simulink model "MinSegShield_Demo_M2V3"  (R2015a)
settings: Solver=FixedStepDiscrete  SolverMode=SingleTasking  StartTime=0.0  StopTime=inf  FixedStep=.03  RelTol=1e-3
libraries: MinSegLibrary_M2V3 x11, arduinolib x5, RASPlib x1
settings Model: SimulationMode=external  ExtModeTrigDuration=2  Creator=Alec  LastModifiedBy=hurstj
settings OptimizationCC: ExpressionDepthLimit=2147483647  OptimizeModelRefInitCode=on  LifeSpan=1
settings DebuggingCC: UnderspecifiedInitializationDetection=Classic  MergeDetectMultiDrivingBlocksExec=none  StateNameClashWarn=warning
settings HardwareCC: ProdBitPerInt=16  ProdBitPerPointer=8  ProdIntDivRoundTo=Zero  ProdEndianess=LittleEndian  ProdWordSize=8  ProdHWDeviceType=Atmel->AVR
settings RTWCC: SystemTargetFile=realtime.tlc  GenerateMakefile=off  TemplateMakefile=realtime.tmf  Description=Real-Time Toolbox  RTWVerbose=off
settings CodeAppCC: MangleLength=10  CustomSymbolStrType=$N$R$M  InternalIdentifier=Classic
settings ERTTargetCC: CombineOutputUpdateFcns=off  ExtMode=on  ExtModeTransport=3  ExtModeMexArgs=0 82 115200  ERTSrcFileBannerTemplate=realtime_code_template.cgt  ERTHdrFileBannerTemplate=realtime_code_template.cgt  ERTDataSrcFileTemplate=realtime_code_template.cgt  ERTDataHdrFileTemplate=realtime_code_template.cgt  ERTCustomFileTemplate=realtime_file_process.tlc

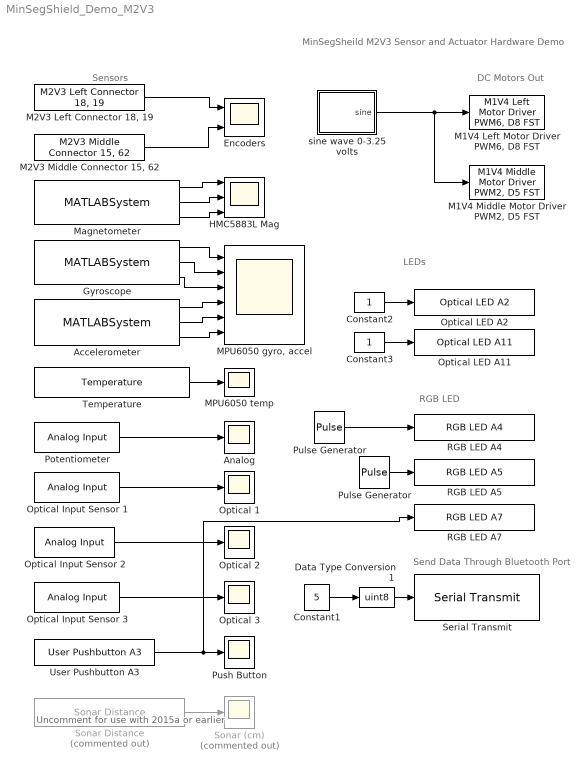
== system MinSegShield_Demo_M2V3 ==
  note: Send Data Through Bluetooth Port
  note: DC Motors Out
  note: Sensors
  note: MinSegSheild M2V3 Sensor and Actuator
      | Hardware Demo
  note: LEDs
  note: RGB LED
  note: Uncomment for use with 2015a or earlier
  Accelerometer : MATLABSystem  System=soMPU6050Accel  SimulateUsing=Code generation
      mask Type: soMPU6050Accel
      mask Display:
      | disp('soMPU6050Accel');
      | port_label('output',1,'xaccel');
      | port_label('output',2,'yaccel');
      | port_label('output',3,'zaccel');
  Analog : Scope
      settings: TimeRange=30  YMin=0  YMax=1000  SaveName=ScopeData6
  Constant1 : Constant  Value=5  SampleTime=-1
  Constant2 : Constant  SampleTime=-1
  Constant3 : Constant  SampleTime=-1
  Data Type Conversion1 : DataTypeConversion  OutDataTypeStr=uint8
  Encoders : Scope  NumInputPorts=2
      settings: TimeRange=20  YMin=-200~-25  YMax=700~250
  Gyroscope : MATLABSystem  System=soMPU6050Gyro  DLPFmode=0
      mask Type: soMPU6050Gyro
      mask Display:
      | disp('soMPU6050Gyro');
      | port_label('output',1,'xvel');
      | port_label('output',2,'yvel');
      | port_label('output',3,'zvel');
  HMC5883L Mag : Scope  NumInputPorts=3
      settings: TimeRange=10  YMin=100~-90~25  YMax=175~30~200  SaveName=ScopeData7
  "M1V4 Left Motor Driver PWM6, D8 FST" : MinSegLibrary_M2V3/M1V4 Left Motor Driver PWM6, D8 FST  Vsupply=3.25
  "M1V4 Middle Motor Driver PWM2, D5 FST" : MinSegLibrary_M2V3/M1V4 Middle Motor Driver PWM2, D5 FST  Vsupply=3.25
  "M2V3 Left Connector 18, 19" : MinSegLibrary_M2V3/M2V3 Left Connector 18, 19  Encoder=1  PinA=19  PinB=18  PWMFSelect=1  PWMTimer=3
  "M2V3 Middle Connector 15, 62" : MinSegLibrary_M2V3/M2V3 Middle Connector 15, 62  Encoder=3  PinA=15  PinB=62  PWMFSelect=1  PWMTimer=3
  "MPU6050 gyro, accel" : Scope  NumInputPorts=6
      settings: TimeRange=10  YMin=-650~-300~-275~100~-400~6000  YMax=-475~-75~-125~800~200~8000
  MPU6050 temp : Scope
      settings: TimeRange=30  YMin=-3750  YMax=-1750  SaveName=ScopeData9
  Magnetometer : MATLABSystem  System=soHMC5883L  SimulateUsing=Code generation
      mask Type: soHMC5883L
      mask Display:
      | disp('soHMC5883L');
      | port_label('output',1,'xmag');
      | port_label('output',2,'ymag');
      | port_label('output',3,'zmag');
  Optical 1 : Scope
      settings: TimeRange=30  YMin=0  YMax=1000  SaveName=ScopeData4
  Optical 2 : Scope
      settings: TimeRange=30  YMin=0  YMax=1000  SaveName=ScopeData3
  Optical 3 : Scope
      settings: TimeRange=30  YMin=0  YMax=1000  SaveName=ScopeData5
  Optical Input Sensor 1 : arduinolib/Analog Input  pinNumber=10  sampleTime=-1  blockPlatform=arduino
  Optical Input Sensor 2 : arduinolib/Analog Input  pinNumber=1  sampleTime=-1  blockPlatform=arduino
  Optical Input Sensor 3 : arduinolib/Analog Input  pinNumber=9  sampleTime=-1  blockPlatform=arduino
  Optical LED A11 : MinSegLibrary_M2V3/Optical LED A11  Pin=11
  Optical LED A2 : MinSegLibrary_M2V3/Optical LED A2  Pin=2
  Potentiometer : arduinolib/Analog Input  pinNumber=0  sampleTime=-1  blockPlatform=arduino
  Pulse Generator : DiscretePulseGenerator  PulseType=Time based  Period=9  PulseWidth=50
  "Pulse Generator " : DiscretePulseGenerator  PulseType=Time based  Period=6  PulseWidth=50
  Push Button : Scope
      settings: TimeRange=30  YMin=0.95  YMax=1.05  SaveName=ScopeData8
  RGB LED A4 : MinSegLibrary_M2V3/RGB LED A4  Pin=4
  RGB LED A5 : MinSegLibrary_M2V3/RGB LED A5  Pin=5
  "RGB LED A7 " : MinSegLibrary_M2V3/RGB LED A7   Pin=7
  Serial Transmit : arduinolib/Serial Transmit  portNumber=2  blockPlatform=arduino
  Sonar (cm) : Scope  Commented=on
      settings: TimeRange=10  YMin=0  YMax=175  SaveName=ScopeData2
  Sonar Distance : MinSegLibrary_M2V3/Sonar Distance  Commented=on  TrigPin=12  EchoPin=11
  Temperature : RASPlib/Temperature  SimulateUsing=Code generation
  User Pushbutton A3 : MinSegLibrary_M2V3/User Pushbutton A3  Pin=3
  sine wave 0-3.25 volts : Subsystem
  wires:
  "M2V3 Left Connector 18, 19"/1 -> Encoders/1
  "M2V3 Middle Connector 15, 62"/1 -> Encoders/2
  Sonar Distance/1 -> Sonar (cm)/1
  Optical Input Sensor 1/1 -> Optical 1/1
  Constant1/1 -> Data Type Conversion1/1
  Data Type Conversion1/1 -> Serial Transmit/1
  Optical Input Sensor 2/1 -> Optical 2/1
  Optical Input Sensor 3/1 -> Optical 3/1
  Potentiometer/1 -> Analog/1
  Magnetometer/2 -> HMC5883L Mag/2
  Magnetometer/3 -> HMC5883L Mag/3
  Gyroscope/1 -> "MPU6050 gyro, accel"/1
  Gyroscope/2 -> "MPU6050 gyro, accel"/2
  Gyroscope/3 -> "MPU6050 gyro, accel"/3
  Accelerometer/3 -> "MPU6050 gyro, accel"/6
  Magnetometer/1 -> HMC5883L Mag/1
  sine wave 0-3.25 volts/1(sine) -> "M1V4 Middle Motor Driver PWM2, D5 FST"/1, "M1V4 Left Motor Driver PWM6, D8 FST"/1
  User Pushbutton A3/1 -> "RGB LED A7 "/1, Push Button/1
  Pulse Generator/1 -> RGB LED A4/1
  "Pulse Generator "/1 -> RGB LED A5/1
  Constant2/1 -> Optical LED A2/1
  Constant3/1 -> Optical LED A11/1
  Accelerometer/1 -> "MPU6050 gyro, accel"/4
  Accelerometer/2 -> "MPU6050 gyro, accel"/5
  Temperature/1 -> MPU6050 temp/1

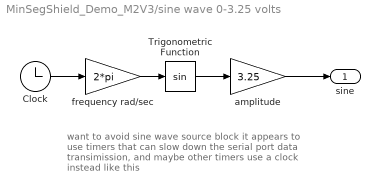
== system MinSegShield_Demo_M2V3/sine wave 0-3.25 volts ==
  note: want to avoid sine wave source block
      | it appears to use timers that can slow down the
      | serial port data transimission, and maybe
      | other timers
      |
      | use a clock instead like this
  Clock : Clock
  Trigonometric Function : Trigonometry
  amplitude : Gain  Gain=3.25
  frequency rad/sec : Gain  Gain=2*pi
  sine : Outport
  wires:
  amplitude/1 -> sine/1
  frequency rad/sec/1 -> Trigonometric Function/1
  Trigonometric Function/1 -> amplitude/1
  Clock/1 -> frequency rad/sec/1
